simulink model "multirate"  (Simulink 6.3)
settings: Solver=FixedStepDiscrete  StartTime=0.0  StopTime=100  FixedStep=1  RelTol=1e-3
InitFcn:
  | %% DSPBuilder Start
  | alt_dspbuilder_update_model(bdroot)
  | %% DSPBuilder End
libraries: allblocks_alteradspbuilder2 x12
settings Model: LastModifiedBy=LKONG  StrictBusMsg=None
settings OptimizationCC: BlockReduction=off  BooleanDataType=off  InlineInvariantSignals=on
settings DebuggingCC: SolverPrmCheckMsg=none
settings HardwareCC: TargetUnknown=on

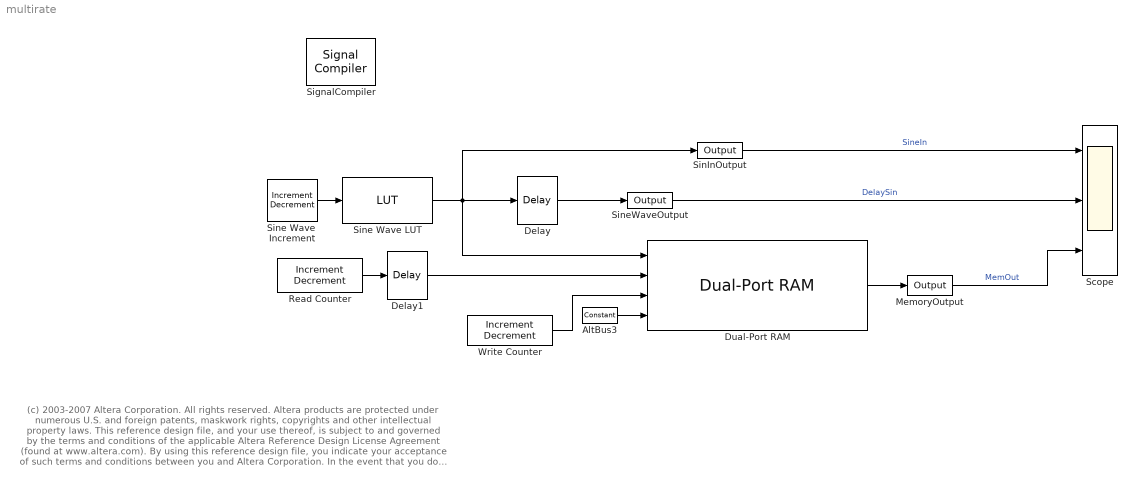
== system multirate ==
  note: (c) 2003-2007 Altera Corporation. All rights reserved.  Altera products are protected under numerous U.S. and foreign patents, maskwork rights, copyrights and other intellectual property laws.
      | This reference design file, and your use thereof, is subject to and governed by the terms and conditions of the applicable Altera Reference Design License Agreement (found at www.altera.com).
      | By using this reference design file, you indicate your acceptance of such terms and conditions between you and Altera Corporation.
      | In the event that you do not agree with such terms and conditions, you may not use the reference design file and please promptly destroy any copies you have made.
      | This reference design file being provided on an "as-is" basis and as an accommodation and therefore all warranties, representations or guarantees of any kind (whether express, implied or statutory)
      | including, without limitation, warranties of merchantability, non-infringement, or fitness for a particular purpose, are specifically disclaimed.
      | By making this reference design file available, Altera expressly does not recommend, suggest or require that this reference design file be used in combination with any other product not provided by Altera
  AltBus3 : allblocks_alteradspbuilder2/Constant  mask_cst=1  BusType=Single Bit  bwl=1  bwr=0  SpecifyClock=off
  Delay : allblocks_alteradspbuilder2/Delay  pipeline=4  ClockPhase=1000  use_ena=off  use_sclr=off
  Delay1 : allblocks_alteradspbuilder2/Delay  pipeline=1  ClockPhase=1  use_ena=off  use_sclr=off
  Dual-Port RAM : allblocks_alteradspbuilder2/Dual-Port RAM  numwords=2^(7)  BusType=Inferred  bwl=8  bwr=0  memory_type=AUTO  ram_type=DualRAM  initialization=Blank  init_file=input.hex  init_array=[0:1:15]  register_outputs=on  use_ena=off  ClockPhase=1
  MemoryOutput : allblocks_alteradspbuilder2/Output  iofile=D:\altera\70\DSPBuilder\DesignExamples\Tutorials\MultiRate\MemoryMultiRate\tb_multirate\multirate_MemoryOutput.capture  BusType=Signed Integer  bwl=10  bwr=0  PORTTYPE=Output
  Read Counter : allblocks_alteradspbuilder2/Increment Decrement  BusType=Unsigned Integer  bwl=7  bwr=0  SpecifyClock=off  clr_value=0  direction=Increment  phase_selection=1  use_ena=off  use_sclr=off
  Scope : Scope  NumInputPorts=3
      settings: TimeRange=50  YMin=-150~-5~-5  YMax=150~5~5
  SignalCompiler : allblocks_alteradspbuilder2/Signal Compiler  DeviceFamily=Stratix III  DeviceName=AUTO  EnableSignalTap=off  SignalTapDepth=128  UseBoardBlock=off  StpUseDefaultClock=on  StpClock=clock
  SinInOutput : allblocks_alteradspbuilder2/Output  iofile=D:\altera\70\DSPBuilder\DesignExamples\Tutorials\MultiRate\MemoryMultiRate\tb_multirate\multirate_SinInOutput.capture  BusType=Signed Integer  bwl=8  bwr=0  PORTTYPE=Output
  Sine Wave  Increment : allblocks_alteradspbuilder2/Increment Decrement  BusType=Unsigned Integer  bwl=6  bwr=0  SpecifyClock=off  clr_value=0  direction=Increment  phase_selection=1  use_ena=off  use_sclr=off
  Sine Wave LUT : allblocks_alteradspbuilder2/LUT  addr_width=6  BusType=Signed Integer  bwl=8  bwr=0  init_array=127*sin( [0:2*pi/(2^6):2*pi] )  use_ena=off  reg_data=off  use_lpm=off  reg_addr=off  ram_type=AUTO
  SineWaveOutput : allblocks_alteradspbuilder2/Output  iofile=D:\altera\70\DSPBuilder\DesignExamples\Tutorials\MultiRate\MemoryMultiRate\tb_multirate\multirate_SineWaveOutput.capture  BusType=Signed Integer  bwl=8  bwr=0  PORTTYPE=Output
  Write Counter : allblocks_alteradspbuilder2/Increment Decrement  BusType=Unsigned Integer  bwl=7  bwr=0  SpecifyClock=off  clr_value=0  direction=Increment  phase_selection=1  use_ena=off  use_sclr=off
  wires:
  Sine Wave LUT/1 -> Delay/1, Dual-Port RAM/1, SinInOutput/1
  Delay/1 -> SineWaveOutput/1
  Dual-Port RAM/1 -> MemoryOutput/1
  AltBus3/1 -> Dual-Port RAM/4
  Read Counter/1 -> Delay1/1
  Sine Wave  Increment/1 -> Sine Wave LUT/1
  MemoryOutput/1 -> Scope/3  "MemOut"
  SineWaveOutput/1 -> Scope/2  "DelaySin"
  SinInOutput/1 -> Scope/1  "SineIn"
  Write Counter/1 -> Dual-Port RAM/3
  Delay1/1 -> Dual-Port RAM/2
